simulink model "MdXX_RspChk"  (R2018b)
settings: Solver=FixedStepDiscrete  StartTime=0.0  StopTime=10.0  FixedStep=0.01  RelTol=1e-3
libraries: OutRspChkLib x20
(part 1 of 2)
settings Model: Creator=sn2xws  LastModifiedBy=sn2xws
settings DataIOCC: SaveFormat=StructureWithTime
settings OptimizationCC: DefaultParameterBehavior=Inlined  EnhancedBackFolding=on  PassReuseOutputArgsAs=Individual arguments  ZeroExternalMemoryAtStartup=off  ZeroInternalMemoryAtStartup=off  OptimizeBlockOrder=speed  DifferentSizesBufferReuse=on  OptimizationCustomize=off
settings DebuggingCC: ParameterTunabilityLossMsg=error
settings ModelReferenceCC: ModelReferenceNumInstancesAllowed=Single
settings SFSimCC: MATLABDynamicMemAlloc=off
settings RTWCC: SystemTargetFile=autosar.tlc  GenCodeOnly=on  TemplateMakefile=ert_default_tmf  Description=AUTOSAR  GenerateReport=on  IncludeHyperlinkInReport=on  LaunchReport=on  GenerateTraceInfo=on  GenerateTraceReport=on  GenerateTraceReportSl=on  GenerateTraceReportSf=on  GenerateTraceReportEml=on
settings CodeAppCC: ForceParamTrailComments=on  IgnoreCustomStorageClasses=off  OperatorAnnotations=on  SimulinkDataObjDesc=on  SFDataObjDesc=on  InsertBlockDesc=on
settings STFCustomTargetCC: TargetLangStandard=C99 (ISO)  MultiwordLength=256  ParMdlRefBuildCompliant=on  CompOptLevelCompliant=on  IncludeMdlTerminateFcn=off  CombineOutputUpdateFcns=on  SuppressErrorStatus=on  ERTCustomFileBanners=on  SupportNonFinite=off  SupportComplex=off  SupportContinuousTime=off  SupportNonInlinedSFcns=off  RemoveResetFunc=on  MATLABClassNameForMDSCustomization=Simulink.SoftwareTarget.ERTCustomization  AutosarCompliant=on  UseToolchainInfoCompliant=on  LookupTableObjectStructAxisOrder=2,1,3,4,...  LUTObjectStructOrderEvenSpacing=Size,Table,Breakpoints  SystemTargetFile=autosar.tlc
settings ERTTargetCC: TargetLangStandard=C99 (ISO)  ConcurrentExecutionCompliant=off  IncludeMdlTerminateFcn=off  SuppressErrorStatus=on  SupportNonFinite=off  SupportComplex=off  ModelStepFunctionPrototypeControlCompliant=off  CPPClassGenCompliant=off  AutosarCompliant=on  LookupTableObjectStructAxisOrder=2,1,3,4,...  LUTObjectStructOrderEvenSpacing=Size,Table,Breakpoints  InlinedParameterPlacement=NonHierarchical  ERTCustomFileTemplate=example_file_process.tlc

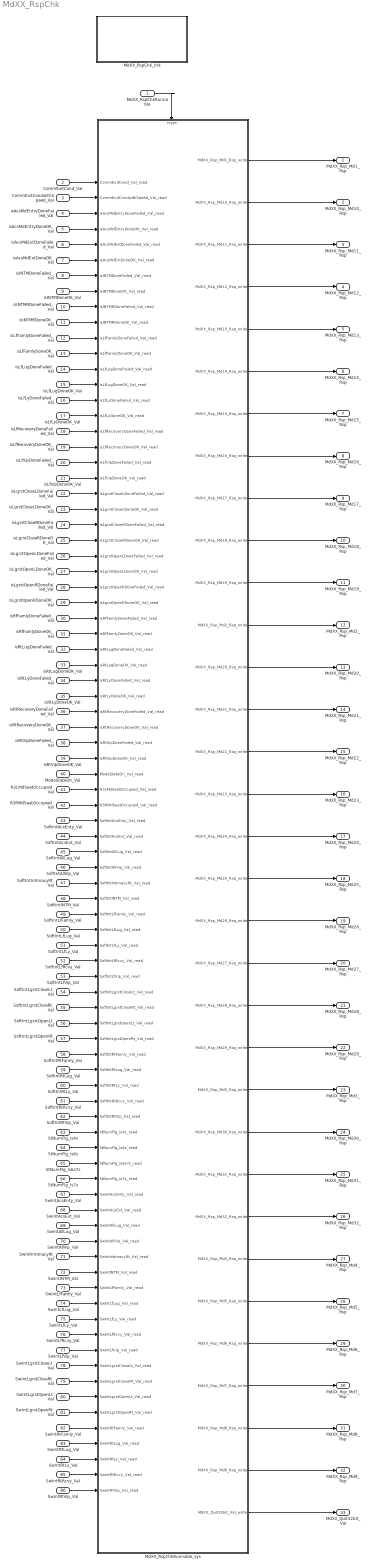
== system MdXX_RspChk ==
  MdXX_RspChkRunnable : Inport  SampleTime=0.01  OutputFunctionCall=on
  CommExitCond_Val : Inport  Port=2  OutDataTypeStr=boolean  PortDimensions=1
  CommExitCondwithSpeed_Val : Inport  Port=3  OutDataTypeStr=boolean  PortDimensions=1
  isAcsMdEntryDoneFailed_Val : Inport  Port=4  OutDataTypeStr=boolean  PortDimensions=1
  isAcsMdEntryDoneOK_Val : Inport  Port=5  OutDataTypeStr=boolean  PortDimensions=1
  isAcsMdExtDoneFailed_Val : Inport  Port=6  OutDataTypeStr=boolean  PortDimensions=1
  isAcsMdExtDoneOK_Val : Inport  Port=7  OutDataTypeStr=boolean  PortDimensions=1
  isINTMDoneFailed_Val : Inport  Port=8  OutDataTypeStr=boolean  PortDimensions=1
  isINTMDoneOK_Val : Inport  Port=9  OutDataTypeStr=boolean  PortDimensions=1
  isINTMRDoneFailed_Val : Inport  Port=10  OutDataTypeStr=boolean  PortDimensions=1
  isINTMRDoneOK_Val : Inport  Port=11  OutDataTypeStr=boolean  PortDimensions=1
  isLfFamlyDoneFailed_Val : Inport  Port=12  OutDataTypeStr=boolean  PortDimensions=1
  isLfFamlyDoneOK_Val : Inport  Port=13  OutDataTypeStr=boolean  PortDimensions=1
  isLfLugDoneFailed_Val : Inport  Port=14  OutDataTypeStr=boolean  PortDimensions=1
  isLfLugDoneOK_Val : Inport  Port=15  OutDataTypeStr=boolean  PortDimensions=1
  isLfLyDoneFailed_Val : Inport  Port=16  OutDataTypeStr=boolean  PortDimensions=1
  isLfLyDoneOK_Val : Inport  Port=17  OutDataTypeStr=boolean  PortDimensions=1
  isLfRecoveryDoneFailed_Val : Inport  Port=18  OutDataTypeStr=boolean  PortDimensions=1
  isLfRecoveryDoneOK_Val : Inport  Port=19  OutDataTypeStr=boolean  PortDimensions=1
  isLfVipDoneFailed_Val : Inport  Port=20  OutDataTypeStr=boolean  PortDimensions=1
  isLfVipDoneOK_Val : Inport  Port=21  OutDataTypeStr=boolean  PortDimensions=1
  isLgrstCloseLDoneFailed_Val : Inport  Port=22  OutDataTypeStr=boolean  PortDimensions=1
  isLgrstCloseLDoneOK_Val : Inport  Port=23  OutDataTypeStr=boolean  PortDimensions=1
  isLgrstCloseRDoneFailed_Val : Inport  Port=24  OutDataTypeStr=boolean  PortDimensions=1
  isLgrstCloseRDoneOK_Val : Inport  Port=25  OutDataTypeStr=boolean  PortDimensions=1
  isLgrstOpenLDoneFailed_Val : Inport  Port=26  OutDataTypeStr=boolean  PortDimensions=1
  isLgrstOpenLDoneOK_Val : Inport  Port=27  OutDataTypeStr=boolean  PortDimensions=1
  isLgrstOpenRDoneFailed_Val : Inport  Port=28  OutDataTypeStr=boolean  PortDimensions=1
  isLgrstOpenRDoneOK_Val : Inport  Port=29  OutDataTypeStr=boolean  PortDimensions=1
  isRfFamlyDoneFailed_Val : Inport  Port=30  OutDataTypeStr=boolean  PortDimensions=1
  isRfFamlyDoneOK_Val : Inport  Port=31  OutDataTypeStr=boolean  PortDimensions=1
  isRtLugDoneFailed_Val : Inport  Port=32  OutDataTypeStr=boolean  PortDimensions=1
  isRtLugDoneOK_Val : Inport  Port=33  OutDataTypeStr=boolean  PortDimensions=1
  isRtLyDoneFailed_Val : Inport  Port=34  OutDataTypeStr=boolean  PortDimensions=1
  isRtLyDoneOK_Val : Inport  Port=35  OutDataTypeStr=boolean  PortDimensions=1
  isRtRecoveryDoneFailed_Val : Inport  Port=36  OutDataTypeStr=boolean  PortDimensions=1
  isRtRecoveryDoneOK_Val : Inport  Port=37  OutDataTypeStr=boolean  PortDimensions=1
  isRtVipDoneFailed_Val : Inport  Port=38  OutDataTypeStr=boolean  PortDimensions=1
  isRtVipDoneOK_Val : Inport  Port=39  OutDataTypeStr=boolean  PortDimensions=1
  ModeStateOn_Val : Inport  Port=40  OutDataTypeStr=boolean  PortDimensions=1
  R3LMdSeatOccupied_Val : Inport  Port=41  OutDataTypeStr=boolean  PortDimensions=1
  R3RMdSeatOccupied_Val : Inport  Port=42  OutDataTypeStr=boolean  PortDimensions=1
  SoftIntAcsEnty_Val : Inport  Port=43  OutDataTypeStr=IntEnable  PortDimensions=1
  SoftIntAcsExt_Val : Inport  Port=44  OutDataTypeStr=IntEnable  PortDimensions=1
  SoftIntAllLug_Val : Inport  Port=45  OutDataTypeStr=IntEnable  PortDimensions=1
  SoftIntAllVip_Val : Inport  Port=46  OutDataTypeStr=IntEnable  PortDimensions=1
  SoftIntIntimacyRt_Val : Inport  Port=47  OutDataTypeStr=IntEnable  PortDimensions=1
  SoftIntINTM_Val : Inport  Port=48  OutDataTypeStr=IntEnable  PortDimensions=1
  SoftIntLfFamly_Val : Inport  Port=49  OutDataTypeStr=IntEnable  PortDimensions=1
  SoftIntLfLug_Val : Inport  Port=50  OutDataTypeStr=IntEnable  PortDimensions=1
  SoftIntLfLy_Val : Inport  Port=51  OutDataTypeStr=IntEnable  PortDimensions=1
  SoftIntLfRcvy_Val : Inport  Port=52  OutDataTypeStr=IntEnable  PortDimensions=1
  SoftIntLfVip_Val : Inport  Port=53  OutDataTypeStr=IntEnable  PortDimensions=1
  SoftIntLgrstCloseLt_Val : Inport  Port=54  OutDataTypeStr=IntEnable  PortDimensions=1
  SoftIntLgrstCloseRt_Val : Inport  Port=55  OutDataTypeStr=IntEnable  PortDimensions=1
  SoftIntLgrstOpenLt_Val : Inport  Port=56  OutDataTypeStr=IntEnable  PortDimensions=1
  SoftIntLgrstOpenRt_Val : Inport  Port=57  OutDataTypeStr=IntEnable  PortDimensions=1
  SoftIntRtFamly_Val : Inport  Port=58  OutDataTypeStr=IntEnable  PortDimensions=1
  SoftIntRtLug_Val : Inport  Port=59  OutDataTypeStr=IntEnable  PortDimensions=1
  SoftIntRtLy_Val : Inport  Port=60  OutDataTypeStr=IntEnable  PortDimensions=1
  SoftIntRtRcvy_Val : Inport  Port=61  OutDataTypeStr=IntEnable  PortDimensions=1
  SoftIntRtVip_Val : Inport  Port=62  OutDataTypeStr=IntEnable  PortDimensions=1
  StNumFlg_Is4s : Inport  Port=63  OutDataTypeStr=boolean  PortDimensions=1
  StNumFlg_Is6s : Inport  Port=64  OutDataTypeStr=boolean  PortDimensions=1
  StNumFlg_Is6s7s : Inport  Port=65  OutDataTypeStr=boolean  PortDimensions=1
  StNumFlg_Is7s : Inport  Port=66  OutDataTypeStr=boolean  PortDimensions=1
  SwIntAcsEnty_Val : Inport  Port=67  OutDataTypeStr=IntEnable  PortDimensions=1
  SwIntAcsExt_Val : Inport  Port=68  OutDataTypeStr=IntEnable  PortDimensions=1
  SwIntAllLug_Val : Inport  Port=69  OutDataTypeStr=IntEnable  PortDimensions=1
  SwIntAllVip_Val : Inport  Port=70  OutDataTypeStr=IntEnable  PortDimensions=1
  SwIntIntimacyRt_Val : Inport  Port=71  OutDataTypeStr=IntEnable  PortDimensions=1
  SwIntINTM_Val : Inport  Port=72  OutDataTypeStr=IntEnable  PortDimensions=1
  SwIntLfFamly_Val : Inport  Port=73  OutDataTypeStr=IntEnable  PortDimensions=1
  SwIntLfLug_Val : Inport  Port=74  OutDataTypeStr=IntEnable  PortDimensions=1
  SwIntLfLy_Val : Inport  Port=75  OutDataTypeStr=IntEnable  PortDimensions=1
  SwIntLfRcvy_Val : Inport  Port=76  OutDataTypeStr=IntEnable  PortDimensions=1
  SwIntLfVip_Val : Inport  Port=77  OutDataTypeStr=IntEnable  PortDimensions=1
  SwIntLgrstCloseLt_Val : Inport  Port=78  OutDataTypeStr=IntEnable  PortDimensions=1
  SwIntLgrstCloseRt_Val : Inport  Port=79  OutDataTypeStr=IntEnable  PortDimensions=1
  SwIntLgrstOpenLt_Val : Inport  Port=80  OutDataTypeStr=IntEnable  PortDimensions=1
  SwIntLgrstOpenRt_Val : Inport  Port=81  OutDataTypeStr=IntEnable  PortDimensions=1
  SwIntRtFamly_Val : Inport  Port=82  OutDataTypeStr=IntEnable  PortDimensions=1
  SwIntRtLug_Val : Inport  Port=83  OutDataTypeStr=IntEnable  PortDimensions=1
  SwIntRtLy_Val : Inport  Port=84  OutDataTypeStr=IntEnable  PortDimensions=1
  SwIntRtRcvy_Val : Inport  Port=85  OutDataTypeStr=IntEnable  PortDimensions=1
  SwIntRtVip_Val : Inport  Port=86  OutDataTypeStr=IntEnable  PortDimensions=1
  MdXX_RspChkRunnable_sys : Subsystem
  MdXX_RspChk_Init : Subsystem
  MdXX_Rsp_Md1_Rsp : Outport  OutDataTypeStr=Enum: MdRspLocal2  PortDimensions=1
  MdXX_Rsp_Md10_Rsp : Outport  Port=2  OutDataTypeStr=Enum: MdRspLocal2  PortDimensions=1
  MdXX_Rsp_Md11_Rsp : Outport  Port=3  OutDataTypeStr=Enum: MdRspLocal2  PortDimensions=1
  MdXX_Rsp_Md12_Rsp : Outport  Port=4  OutDataTypeStr=Enum: MdRspLocal2  PortDimensions=1
  MdXX_Rsp_Md13_Rsp : Outport  Port=5  OutDataTypeStr=Enum: MdRspLocal2  PortDimensions=1
  MdXX_Rsp_Md14_Rsp : Outport  Port=6  OutDataTypeStr=Enum: MdRspLocal2  PortDimensions=1
  MdXX_Rsp_Md15_Rsp : Outport  Port=7  OutDataTypeStr=Enum: MdRspLocal2  PortDimensions=1
  MdXX_Rsp_Md16_Rsp : Outport  Port=8  OutDataTypeStr=Enum: MdRspLocal2  PortDimensions=1
  MdXX_Rsp_Md17_Rsp : Outport  Port=9  OutDataTypeStr=Enum: MdRspLocal2  PortDimensions=1
  MdXX_Rsp_Md18_Rsp : Outport  Port=10  OutDataTypeStr=Enum: MdRspLocal2  PortDimensions=1
  MdXX_Rsp_Md19_Rsp : Outport  Port=11  OutDataTypeStr=Enum: MdRspLocal2  PortDimensions=1
  MdXX_Rsp_Md2_Rsp : Outport  Port=12  OutDataTypeStr=Enum: MdRspLocal2  PortDimensions=1
  MdXX_Rsp_Md20_Rsp : Outport  Port=13  OutDataTypeStr=Enum: MdRspLocal2  PortDimensions=1
  MdXX_Rsp_Md21_Rsp : Outport  Port=14  OutDataTypeStr=Enum: MdRspLocal2  PortDimensions=1
  MdXX_Rsp_Md22_Rsp : Outport  Port=15  OutDataTypeStr=Enum: MdRspLocal2  PortDimensions=1
  MdXX_Rsp_Md23_Rsp : Outport  Port=16  OutDataTypeStr=Enum: MdRspLocal2  PortDimensions=1
  MdXX_Rsp_Md24_Rsp : Outport  Port=17  OutDataTypeStr=Enum: MdRspLocal2  PortDimensions=1
  MdXX_Rsp_Md25_Rsp : Outport  Port=18  OutDataTypeStr=Enum: MdRspLocal2  PortDimensions=1
  MdXX_Rsp_Md26_Rsp : Outport  Port=19  OutDataTypeStr=Enum: MdRspLocal2  PortDimensions=1
  MdXX_Rsp_Md27_Rsp : Outport  Port=20  OutDataTypeStr=Enum: MdRspLocal2  PortDimensions=1
  MdXX_Rsp_Md28_Rsp : Outport  Port=21  OutDataTypeStr=Enum: MdRspLocal2  PortDimensions=1
  MdXX_Rsp_Md29_Rsp : Outport  Port=22  OutDataTypeStr=Enum: MdRspLocal2  PortDimensions=1
  MdXX_Rsp_Md3_Rsp : Outport  Port=23  OutDataTypeStr=Enum: MdRspLocal2  PortDimensions=1
  MdXX_Rsp_Md30_Rsp : Outport  Port=24  OutDataTypeStr=Enum: MdRspLocal2  PortDimensions=1
  MdXX_Rsp_Md31_Rsp : Outport  Port=25  OutDataTypeStr=Enum: MdRspLocal2  PortDimensions=1
  MdXX_Rsp_Md32_Rsp : Outport  Port=26  OutDataTypeStr=Enum: MdRspLocal2  PortDimensions=1
  MdXX_Rsp_Md4_Rsp : Outport  Port=27  OutDataTypeStr=Enum: MdRspLocal2  PortDimensions=1
  MdXX_Rsp_Md5_Rsp : Outport  Port=28  OutDataTypeStr=Enum: MdRspLocal2  PortDimensions=1
  MdXX_Rsp_Md6_Rsp : Outport  Port=29  OutDataTypeStr=Enum: MdRspLocal2  PortDimensions=1
  MdXX_Rsp_Md7_Rsp : Outport  Port=30  OutDataTypeStr=Enum: MdRspLocal2  PortDimensions=1
  MdXX_Rsp_Md8_Rsp : Outport  Port=31  OutDataTypeStr=Enum: MdRspLocal2  PortDimensions=1
  MdXX_Rsp_Md9_Rsp : Outport  Port=32  OutDataTypeStr=Enum: MdRspLocal2  PortDimensions=1
  MdXX_Quit32bit_Val : Outport  Port=33  OutDataTypeStr=uint32  PortDimensions=1
  wires:
  CommExitCond_Val/1 -> MdXX_RspChkRunnable_sys/1(CommExitCond_Val_read)
  CommExitCondwithSpeed_Val/1 -> MdXX_RspChkRunnable_sys/2(CommExitCondwithSpeed_Val_read)
  isAcsMdEntryDoneFailed_Val/1 -> MdXX_RspChkRunnable_sys/3(isAcsMdEntryDoneFailed_Val_read)
  isAcsMdEntryDoneOK_Val/1 -> MdXX_RspChkRunnable_sys/4(isAcsMdEntryDoneOK_Val_read)
  isAcsMdExtDoneFailed_Val/1 -> MdXX_RspChkRunnable_sys/5(isAcsMdExtDoneFailed_Val_read)
  isAcsMdExtDoneOK_Val/1 -> MdXX_RspChkRunnable_sys/6(isAcsMdExtDoneOK_Val_read)
  isINTMDoneFailed_Val/1 -> MdXX_RspChkRunnable_sys/7(isINTMDoneFailed_Val_read)
  isINTMDoneOK_Val/1 -> MdXX_RspChkRunnable_sys/8(isINTMDoneOK_Val_read)
  isINTMRDoneFailed_Val/1 -> MdXX_RspChkRunnable_sys/9(isINTMRDoneFailed_Val_read)
  isINTMRDoneOK_Val/1 -> MdXX_RspChkRunnable_sys/10(isINTMRDoneOK_Val_read)
  isLfFamlyDoneFailed_Val/1 -> MdXX_RspChkRunnable_sys/11(isLfFamlyDoneFailed_Val_read)
  isLfFamlyDoneOK_Val/1 -> MdXX_RspChkRunnable_sys/12(isLfFamlyDoneOK_Val_read)
  isLfLugDoneFailed_Val/1 -> MdXX_RspChkRunnable_sys/13(isLfLugDoneFailed_Val_read)
  isLfLugDoneOK_Val/1 -> MdXX_RspChkRunnable_sys/14(isLfLugDoneOK_Val_read)
  isLfLyDoneFailed_Val/1 -> MdXX_RspChkRunnable_sys/15(isLfLyDoneFailed_Val_read)
  isLfLyDoneOK_Val/1 -> MdXX_RspChkRunnable_sys/16(isLfLyDoneOK_Val_read)
  isLfRecoveryDoneFailed_Val/1 -> MdXX_RspChkRunnable_sys/17(isLfRecoveryDoneFailed_Val_read)
  isLfRecoveryDoneOK_Val/1 -> MdXX_RspChkRunnable_sys/18(isLfRecoveryDoneOK_Val_read)
  isLfVipDoneFailed_Val/1 -> MdXX_RspChkRunnable_sys/19(isLfVipDoneFailed_Val_read)
  isLfVipDoneOK_Val/1 -> MdXX_RspChkRunnable_sys/20(isLfVipDoneOK_Val_read)
  isLgrstCloseLDoneFailed_Val/1 -> MdXX_RspChkRunnable_sys/21(isLgrstCloseLDoneFailed_Val_read)
  isLgrstCloseLDoneOK_Val/1 -> MdXX_RspChkRunnable_sys/22(isLgrstCloseLDoneOK_Val_read)
  isLgrstCloseRDoneFailed_Val/1 -> MdXX_RspChkRunnable_sys/23(isLgrstCloseRDoneFailed_Val_read)
  isLgrstCloseRDoneOK_Val/1 -> MdXX_RspChkRunnable_sys/24(isLgrstCloseRDoneOK_Val_read)
  isLgrstOpenLDoneFailed_Val/1 -> MdXX_RspChkRunnable_sys/25(isLgrstOpenLDoneFailed_Val_read)
  isLgrstOpenLDoneOK_Val/1 -> MdXX_RspChkRunnable_sys/26(isLgrstOpenLDoneOK_Val_read)
  isLgrstOpenRDoneFailed_Val/1 -> MdXX_RspChkRunnable_sys/27(isLgrstOpenRDoneFailed_Val_read)
  isLgrstOpenRDoneOK_Val/1 -> MdXX_RspChkRunnable_sys/28(isLgrstOpenRDoneOK_Val_read)
  isRfFamlyDoneFailed_Val/1 -> MdXX_RspChkRunnable_sys/29(isRfFamlyDoneFailed_Val_read)
  isRfFamlyDoneOK_Val/1 -> MdXX_RspChkRunnable_sys/30(isRfFamlyDoneOK_Val_read)
  isRtLugDoneFailed_Val/1 -> MdXX_RspChkRunnable_sys/31(isRtLugDoneFailed_Val_read)
  isRtLugDoneOK_Val/1 -> MdXX_RspChkRunnable_sys/32(isRtLugDoneOK_Val_read)
  isRtLyDoneFailed_Val/1 -> MdXX_RspChkRunnable_sys/33(isRtLyDoneFailed_Val_read)
  isRtLyDoneOK_Val/1 -> MdXX_RspChkRunnable_sys/34(isRtLyDoneOK_Val_read)
  isRtRecoveryDoneFailed_Val/1 -> MdXX_RspChkRunnable_sys/35(isRtRecoveryDoneFailed_Val_read)
  isRtRecoveryDoneOK_Val/1 -> MdXX_RspChkRunnable_sys/36(isRtRecoveryDoneOK_Val_read)
  isRtVipDoneFailed_Val/1 -> MdXX_RspChkRunnable_sys/37(isRtVipDoneFailed_Val_read)
  isRtVipDoneOK_Val/1 -> MdXX_RspChkRunnable_sys/38(isRtVipDoneOK_Val_read)
  ModeStateOn_Val/1 -> MdXX_RspChkRunnable_sys/39(ModeStateOn_Val_read)
  R3LMdSeatOccupied_Val/1 -> MdXX_RspChkRunnable_sys/40(R3LMdSeatOccupied_Val_read)
  R3RMdSeatOccupied_Val/1 -> MdXX_RspChkRunnable_sys/41(R3RMdSeatOccupied_Val_read)
  SoftIntAcsEnty_Val/1 -> MdXX_RspChkRunnable_sys/42(SoftIntAcsEnty_Val_read)
  SoftIntAcsExt_Val/1 -> MdXX_RspChkRunnable_sys/43(SoftIntAcsExt_Val_read)
  SoftIntAllLug_Val/1 -> MdXX_RspChkRunnable_sys/44(SoftIntAllLug_Val_read)
  SoftIntAllVip_Val/1 -> MdXX_RspChkRunnable_sys/45(SoftIntAllVip_Val_read)
  SoftIntIntimacyRt_Val/1 -> MdXX_RspChkRunnable_sys/46(SoftIntIntimacyRt_Val_read)
  SoftIntINTM_Val/1 -> MdXX_RspChkRunnable_sys/47(SoftIntINTM_Val_read)
  SoftIntLfFamly_Val/1 -> MdXX_RspChkRunnable_sys/48(SoftIntLfFamly_Val_read)
  SoftIntLfLug_Val/1 -> MdXX_RspChkRunnable_sys/49(SoftIntLfLug_Val_read)
  SoftIntLfLy_Val/1 -> MdXX_RspChkRunnable_sys/50(SoftIntLfLy_Val_read)
  SoftIntLfRcvy_Val/1 -> MdXX_RspChkRunnable_sys/51(SoftIntLfRcvy_Val_read)
  SoftIntLfVip_Val/1 -> MdXX_RspChkRunnable_sys/52(SoftIntLfVip_Val_read)
  SoftIntLgrstCloseLt_Val/1 -> MdXX_RspChkRunnable_sys/53(SoftIntLgrstCloseLt_Val_read)
  SoftIntLgrstCloseRt_Val/1 -> MdXX_RspChkRunnable_sys/54(SoftIntLgrstCloseRt_Val_read)
  SoftIntLgrstOpenLt_Val/1 -> MdXX_RspChkRunnable_sys/55(SoftIntLgrstOpenLt_Val_read)
  SoftIntLgrstOpenRt_Val/1 -> MdXX_RspChkRunnable_sys/56(SoftIntLgrstOpenRt_Val_read)
  SoftIntRtFamly_Val/1 -> MdXX_RspChkRunnable_sys/57(SoftIntRtFamly_Val_read)
  SoftIntRtLug_Val/1 -> MdXX_RspChkRunnable_sys/58(SoftIntRtLug_Val_read)
  SoftIntRtLy_Val/1 -> MdXX_RspChkRunnable_sys/59(SoftIntRtLy_Val_read)
  SoftIntRtRcvy_Val/1 -> MdXX_RspChkRunnable_sys/60(SoftIntRtRcvy_Val_read)
  SoftIntRtVip_Val/1 -> MdXX_RspChkRunnable_sys/61(SoftIntRtVip_Val_read)
  StNumFlg_Is4s/1 -> MdXX_RspChkRunnable_sys/62(StNumFlg_Is4s_read)
  StNumFlg_Is6s/1 -> MdXX_RspChkRunnable_sys/63(StNumFlg_Is6s_read)
  StNumFlg_Is6s7s/1 -> MdXX_RspChkRunnable_sys/64(StNumFlg_Is6s7s_read)
  StNumFlg_Is7s/1 -> MdXX_RspChkRunnable_sys/65(StNumFlg_Is7s_read)
  SwIntAcsEnty_Val/1 -> MdXX_RspChkRunnable_sys/66(SwIntAcsEnty_Val_read)
  SwIntAcsExt_Val/1 -> MdXX_RspChkRunnable_sys/67(SwIntAcsExt_Val_read)
  SwIntAllLug_Val/1 -> MdXX_RspChkRunnable_sys/68(SwIntAllLug_Val_read)
  SwIntAllVip_Val/1 -> MdXX_RspChkRunnable_sys/69(SwIntAllVip_Val_read)
  SwIntIntimacyRt_Val/1 -> MdXX_RspChkRunnable_sys/70(SwIntIntimacyRt_Val_read)
  SwIntINTM_Val/1 -> MdXX_RspChkRunnable_sys/71(SwIntINTM_Val_read)
  SwIntLfFamly_Val/1 -> MdXX_RspChkRunnable_sys/72(SwIntLfFamly_Val_read)
  SwIntLfLug_Val/1 -> MdXX_RspChkRunnable_sys/73(SwIntLfLug_Val_read)
  SwIntLfLy_Val/1 -> MdXX_RspChkRunnable_sys/74(SwIntLfLy_Val_read)
  SwIntLfRcvy_Val/1 -> MdXX_RspChkRunnable_sys/75(SwIntLfRcvy_Val_read)
  SwIntLfVip_Val/1 -> MdXX_RspChkRunnable_sys/76(SwIntLfVip_Val_read)
  SwIntLgrstCloseLt_Val/1 -> MdXX_RspChkRunnable_sys/77(SwIntLgrstCloseLt_Val_read)
  SwIntLgrstCloseRt_Val/1 -> MdXX_RspChkRunnable_sys/78(SwIntLgrstCloseRt_Val_read)
  SwIntLgrstOpenLt_Val/1 -> MdXX_RspChkRunnable_sys/79(SwIntLgrstOpenLt_Val_read)
  SwIntLgrstOpenRt_Val/1 -> MdXX_RspChkRunnable_sys/80(SwIntLgrstOpenRt_Val_read)
  SwIntRtFamly_Val/1 -> MdXX_RspChkRunnable_sys/81(SwIntRtFamly_Val_read)
  SwIntRtLug_Val/1 -> MdXX_RspChkRunnable_sys/82(SwIntRtLug_Val_read)
  SwIntRtLy_Val/1 -> MdXX_RspChkRunnable_sys/83(SwIntRtLy_Val_read)
  SwIntRtRcvy_Val/1 -> MdXX_RspChkRunnable_sys/84(SwIntRtRcvy_Val_read)
  SwIntRtVip_Val/1 -> MdXX_RspChkRunnable_sys/85(SwIntRtVip_Val_read)
  MdXX_RspChkRunnable_sys/1(MdXX_Rsp_Md1_Rsp_write) -> MdXX_Rsp_Md1_Rsp/1
  MdXX_RspChkRunnable_sys/2(MdXX_Rsp_Md10_Rsp_write) -> MdXX_Rsp_Md10_Rsp/1
  MdXX_RspChkRunnable_sys/3(MdXX_Rsp_Md11_Rsp_write) -> MdXX_Rsp_Md11_Rsp/1
  MdXX_RspChkRunnable_sys/4(MdXX_Rsp_Md12_Rsp_write) -> MdXX_Rsp_Md12_Rsp/1
  MdXX_RspChkRunnable_sys/5(MdXX_Rsp_Md13_Rsp_write) -> MdXX_Rsp_Md13_Rsp/1
  MdXX_RspChkRunnable_sys/6(MdXX_Rsp_Md14_Rsp_write) -> MdXX_Rsp_Md14_Rsp/1
  MdXX_RspChkRunnable_sys/7(MdXX_Rsp_Md15_Rsp_write) -> MdXX_Rsp_Md15_Rsp/1
  MdXX_RspChkRunnable_sys/8(MdXX_Rsp_Md16_Rsp_write) -> MdXX_Rsp_Md16_Rsp/1
  MdXX_RspChkRunnable_sys/9(MdXX_Rsp_Md17_Rsp_write) -> MdXX_Rsp_Md17_Rsp/1
  MdXX_RspChkRunnable_sys/10(MdXX_Rsp_Md18_Rsp_write) -> MdXX_Rsp_Md18_Rsp/1
  MdXX_RspChkRunnable_sys/11(MdXX_Rsp_Md19_Rsp_write) -> MdXX_Rsp_Md19_Rsp/1
  MdXX_RspChkRunnable_sys/12(MdXX_Rsp_Md2_Rsp_write) -> MdXX_Rsp_Md2_Rsp/1
  MdXX_RspChkRunnable_sys/13(MdXX_Rsp_Md20_Rsp_write) -> MdXX_Rsp_Md20_Rsp/1
  MdXX_RspChkRunnable_sys/14(MdXX_Rsp_Md21_Rsp_write) -> MdXX_Rsp_Md21_Rsp/1
  MdXX_RspChkRunnable_sys/15(MdXX_Rsp_Md22_Rsp_write) -> MdXX_Rsp_Md22_Rsp/1
  MdXX_RspChkRunnable_sys/16(MdXX_Rsp_Md23_Rsp_write) -> MdXX_Rsp_Md23_Rsp/1
  MdXX_RspChkRunnable_sys/17(MdXX_Rsp_Md24_Rsp_write) -> MdXX_Rsp_Md24_Rsp/1
  MdXX_RspChkRunnable_sys/18(MdXX_Rsp_Md25_Rsp_write) -> MdXX_Rsp_Md25_Rsp/1
  MdXX_RspChkRunnable_sys/19(MdXX_Rsp_Md26_Rsp_write) -> MdXX_Rsp_Md26_Rsp/1
  MdXX_RspChkRunnable_sys/20(MdXX_Rsp_Md27_Rsp_write) -> MdXX_Rsp_Md27_Rsp/1
  MdXX_RspChkRunnable_sys/21(MdXX_Rsp_Md28_Rsp_write) -> MdXX_Rsp_Md28_Rsp/1
  MdXX_RspChkRunnable_sys/22(MdXX_Rsp_Md29_Rsp_write) -> MdXX_Rsp_Md29_Rsp/1
  MdXX_RspChkRunnable_sys/23(MdXX_Rsp_Md3_Rsp_write) -> MdXX_Rsp_Md3_Rsp/1
  MdXX_RspChkRunnable_sys/24(MdXX_Rsp_Md30_Rsp_write) -> MdXX_Rsp_Md30_Rsp/1
  MdXX_RspChkRunnable_sys/25(MdXX_Rsp_Md31_Rsp_write) -> MdXX_Rsp_Md31_Rsp/1
  MdXX_RspChkRunnable_sys/26(MdXX_Rsp_Md32_Rsp_write) -> MdXX_Rsp_Md32_Rsp/1
  MdXX_RspChkRunnable_sys/27(MdXX_Rsp_Md4_Rsp_write) -> MdXX_Rsp_Md4_Rsp/1
  MdXX_RspChkRunnable_sys/28(MdXX_Rsp_Md5_Rsp_write) -> MdXX_Rsp_Md5_Rsp/1
  MdXX_RspChkRunnable_sys/29(MdXX_Rsp_Md6_Rsp_write) -> MdXX_Rsp_Md6_Rsp/1
  MdXX_RspChkRunnable_sys/30(MdXX_Rsp_Md7_Rsp_write) -> MdXX_Rsp_Md7_Rsp/1
  MdXX_RspChkRunnable_sys/31(MdXX_Rsp_Md8_Rsp_write) -> MdXX_Rsp_Md8_Rsp/1
  MdXX_RspChkRunnable_sys/32(MdXX_Rsp_Md9_Rsp_write) -> MdXX_Rsp_Md9_Rsp/1
  MdXX_RspChkRunnable_sys/33(MdXX_Quit32bit_Val_write) -> MdXX_Quit32bit_Val/1
  MdXX_RspChkRunnable/1 -> MdXX_RspChkRunnable_sys/Trigger

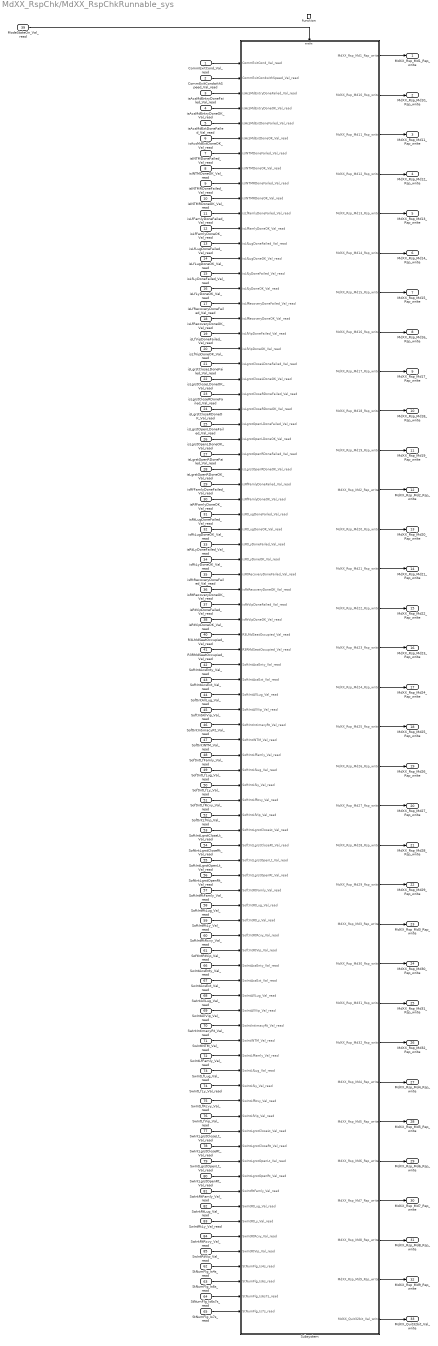
== system MdXX_RspChk/MdXX_RspChkRunnable_sys ==
  CommExitCond_Val_read : Inport
  CommExitCondwithSpeed_Val_read : Inport  Port=2
  isAcsMdEntryDoneFailed_Val_read : Inport  Port=3
  isAcsMdEntryDoneOK_Val_read : Inport  Port=4
  isAcsMdExtDoneFailed_Val_read : Inport  Port=5
  isAcsMdExtDoneOK_Val_read : Inport  Port=6
  isINTMDoneFailed_Val_read : Inport  Port=7
  isINTMDoneOK_Val_read : Inport  Port=8
  isINTMRDoneFailed_Val_read : Inport  Port=9
  isINTMRDoneOK_Val_read : Inport  Port=10
  isLfFamlyDoneFailed_Val_read : Inport  Port=11
  isLfFamlyDoneOK_Val_read : Inport  Port=12
  isLfLugDoneFailed_Val_read : Inport  Port=13
  isLfLugDoneOK_Val_read : Inport  Port=14
  isLfLyDoneFailed_Val_read : Inport  Port=15
  isLfLyDoneOK_Val_read : Inport  Port=16
  isLfRecoveryDoneFailed_Val_read : Inport  Port=17
  isLfRecoveryDoneOK_Val_read : Inport  Port=18
  isLfVipDoneFailed_Val_read : Inport  Port=19
  isLfVipDoneOK_Val_read : Inport  Port=20
  isLgrstCloseLDoneFailed_Val_read : Inport  Port=21
  isLgrstCloseLDoneOK_Val_read : Inport  Port=22
  isLgrstCloseRDoneFailed_Val_read : Inport  Port=23
  isLgrstCloseRDoneOK_Val_read : Inport  Port=24
  isLgrstOpenLDoneFailed_Val_read : Inport  Port=25
  isLgrstOpenLDoneOK_Val_read : Inport  Port=26
  isLgrstOpenRDoneFailed_Val_read : Inport  Port=27
  isLgrstOpenRDoneOK_Val_read : Inport  Port=28
  isRfFamlyDoneFailed_Val_read : Inport  Port=29
  isRfFamlyDoneOK_Val_read : Inport  Port=30
  isRtLugDoneFailed_Val_read : Inport  Port=31
  isRtLugDoneOK_Val_read : Inport  Port=32
  isRtLyDoneFailed_Val_read : Inport  Port=33
  isRtLyDoneOK_Val_read : Inport  Port=34
  isRtRecoveryDoneFailed_Val_read : Inport  Port=35
  isRtRecoveryDoneOK_Val_read : Inport  Port=36
  isRtVipDoneFailed_Val_read : Inport  Port=37
  isRtVipDoneOK_Val_read : Inport  Port=38
  ModeStateOn_Val_read : Inport  Port=39
  R3LMdSeatOccupied_Val_read : Inport  Port=40
  R3RMdSeatOccupied_Val_read : Inport  Port=41
  SoftIntAcsEnty_Val_read : Inport  Port=42
  SoftIntAcsExt_Val_read : Inport  Port=43
  SoftIntAllLug_Val_read : Inport  Port=44
  SoftIntAllVip_Val_read : Inport  Port=45
  SoftIntIntimacyRt_Val_read : Inport  Port=46
  SoftIntINTM_Val_read : Inport  Port=47
  SoftIntLfFamly_Val_read : Inport  Port=48
  SoftIntLfLug_Val_read : Inport  Port=49
  SoftIntLfLy_Val_read : Inport  Port=50
  SoftIntLfRcvy_Val_read : Inport  Port=51
  SoftIntLfVip_Val_read : Inport  Port=52
  SoftIntLgrstCloseLt_Val_read : Inport  Port=53
  SoftIntLgrstCloseRt_Val_read : Inport  Port=54
  SoftIntLgrstOpenLt_Val_read : Inport  Port=55
  SoftIntLgrstOpenRt_Val_read : Inport  Port=56
  SoftIntRtFamly_Val_read : Inport  Port=57
  SoftIntRtLug_Val_read : Inport  Port=58
  SoftIntRtLy_Val_read : Inport  Port=59
  SoftIntRtRcvy_Val_read : Inport  Port=60
  SoftIntRtVip_Val_read : Inport  Port=61
  StNumFlg_Is4s_read : Inport  Port=62
  StNumFlg_Is6s_read : Inport  Port=63
  StNumFlg_Is6s7s_read : Inport  Port=64
  StNumFlg_Is7s_read : Inport  Port=65
  SwIntAcsEnty_Val_read : Inport  Port=66
  SwIntAcsExt_Val_read : Inport  Port=67
  SwIntAllLug_Val_read : Inport  Port=68
  SwIntAllVip_Val_read : Inport  Port=69
  SwIntIntimacyRt_Val_read : Inport  Port=70
  SwIntINTM_Val_read : Inport  Port=71
  SwIntLfFamly_Val_read : Inport  Port=72
  SwIntLfLug_Val_read : Inport  Port=73
  SwIntLfLy_Val_read : Inport  Port=74
  SwIntLfRcvy_Val_read : Inport  Port=75
  SwIntLfVip_Val_read : Inport  Port=76
  SwIntLgrstCloseLt_Val_read : Inport  Port=77
  SwIntLgrstCloseRt_Val_read : Inport  Port=78
  SwIntLgrstOpenLt_Val_read : Inport  Port=79
  SwIntLgrstOpenRt_Val_read : Inport  Port=80
  SwIntRtFamly_Val_read : Inport  Port=81
  SwIntRtLug_Val_read : Inport  Port=82
  SwIntRtLy_Val_read : Inport  Port=83
  SwIntRtRcvy_Val_read : Inport  Port=84
  SwIntRtVip_Val_read : Inport  Port=85
  function : TriggerPort  TriggerType=function-call  VariantControl=(inherit)  SampleTimeType=periodic  SampleTime=-1
  Subsystem : Subsystem
  MdXX_Rsp_Md1_Rsp_write : Outport
      settings: EnsureOutportIsVirtual=on
  MdXX_Rsp_Md10_Rsp_write : Outport  Port=2
      settings: EnsureOutportIsVirtual=on
  MdXX_Rsp_Md11_Rsp_write : Outport  Port=3
      settings: EnsureOutportIsVirtual=on
  MdXX_Rsp_Md12_Rsp_write : Outport  Port=4
      settings: EnsureOutportIsVirtual=on
  MdXX_Rsp_Md13_Rsp_write : Outport  Port=5
      settings: EnsureOutportIsVirtual=on
  MdXX_Rsp_Md14_Rsp_write : Outport  Port=6
      settings: EnsureOutportIsVirtual=on
  MdXX_Rsp_Md15_Rsp_write : Outport  Port=7
      settings: EnsureOutportIsVirtual=on
  MdXX_Rsp_Md16_Rsp_write : Outport  Port=8
      settings: EnsureOutportIsVirtual=on
  MdXX_Rsp_Md17_Rsp_write : Outport  Port=9
      settings: EnsureOutportIsVirtual=on
  MdXX_Rsp_Md18_Rsp_write : Outport  Port=10
      settings: EnsureOutportIsVirtual=on
  MdXX_Rsp_Md19_Rsp_write : Outport  Port=11
      settings: EnsureOutportIsVirtual=on
  MdXX_Rsp_Md2_Rsp_write : Outport  Port=12
      settings: EnsureOutportIsVirtual=on
  MdXX_Rsp_Md20_Rsp_write : Outport  Port=13
      settings: EnsureOutportIsVirtual=on
  MdXX_Rsp_Md21_Rsp_write : Outport  Port=14
      settings: EnsureOutportIsVirtual=on
  MdXX_Rsp_Md22_Rsp_write : Outport  Port=15
      settings: EnsureOutportIsVirtual=on
  MdXX_Rsp_Md23_Rsp_write : Outport  Port=16
      settings: EnsureOutportIsVirtual=on
  MdXX_Rsp_Md24_Rsp_write : Outport  Port=17
      settings: EnsureOutportIsVirtual=on
  MdXX_Rsp_Md25_Rsp_write : Outport  Port=18
      settings: EnsureOutportIsVirtual=on
  MdXX_Rsp_Md26_Rsp_write : Outport  Port=19
      settings: EnsureOutportIsVirtual=on
  MdXX_Rsp_Md27_Rsp_write : Outport  Port=20
      settings: EnsureOutportIsVirtual=on
  MdXX_Rsp_Md28_Rsp_write : Outport  Port=21
      settings: EnsureOutportIsVirtual=on
  MdXX_Rsp_Md29_Rsp_write : Outport  Port=22
      settings: EnsureOutportIsVirtual=on
  MdXX_Rsp_Md3_Rsp_write : Outport  Port=23
      settings: EnsureOutportIsVirtual=on
  MdXX_Rsp_Md30_Rsp_write : Outport  Port=24
      settings: EnsureOutportIsVirtual=on
  MdXX_Rsp_Md31_Rsp_write : Outport  Port=25
      settings: EnsureOutportIsVirtual=on
  MdXX_Rsp_Md32_Rsp_write : Outport  Port=26
      settings: EnsureOutportIsVirtual=on
  MdXX_Rsp_Md4_Rsp_write : Outport  Port=27
      settings: EnsureOutportIsVirtual=on
  MdXX_Rsp_Md5_Rsp_write : Outport  Port=28
      settings: EnsureOutportIsVirtual=on
  MdXX_Rsp_Md6_Rsp_write : Outport  Port=29
      settings: EnsureOutportIsVirtual=on
  MdXX_Rsp_Md7_Rsp_write : Outport  Port=30
      settings: EnsureOutportIsVirtual=on
  MdXX_Rsp_Md8_Rsp_write : Outport  Port=31
      settings: EnsureOutportIsVirtual=on
  MdXX_Rsp_Md9_Rsp_write : Outport  Port=32
      settings: EnsureOutportIsVirtual=on
  MdXX_Quit32bit_Val_write : Outport  Port=33
      settings: EnsureOutportIsVirtual=on
  wires:
  ModeStateOn_Val_read/1 -> Subsystem/Enable
  CommExitCond_Val_read/1 -> Subsystem/1(CommExitCond_Val_read)
  CommExitCondwithSpeed_Val_read/1 -> Subsystem/2(CommExitCondwithSpeed_Val_read)
  isAcsMdEntryDoneFailed_Val_read/1 -> Subsystem/3(isAcsMdEntryDoneFailed_Val_read)
  isAcsMdEntryDoneOK_Val_read/1 -> Subsystem/4(isAcsMdEntryDoneOK_Val_read)
  isAcsMdExtDoneFailed_Val_read/1 -> Subsystem/5(isAcsMdExtDoneFailed_Val_read)
  isAcsMdExtDoneOK_Val_read/1 -> Subsystem/6(isAcsMdExtDoneOK_Val_read)
  isINTMDoneFailed_Val_read/1 -> Subsystem/7(isINTMDoneFailed_Val_read)
  isINTMDoneOK_Val_read/1 -> Subsystem/8(isINTMDoneOK_Val_read)
  isINTMRDoneFailed_Val_read/1 -> Subsystem/9(isINTMRDoneFailed_Val_read)
  isINTMRDoneOK_Val_read/1 -> Subsystem/10(isINTMRDoneOK_Val_read)
  isLfFamlyDoneFailed_Val_read/1 -> Subsystem/11(isLfFamlyDoneFailed_Val_read)
  isLfFamlyDoneOK_Val_read/1 -> Subsystem/12(isLfFamlyDoneOK_Val_read)
  isLfLugDoneFailed_Val_read/1 -> Subsystem/13(isLfLugDoneFailed_Val_read)
  isLfLugDoneOK_Val_read/1 -> Subsystem/14(isLfLugDoneOK_Val_read)
  isLfLyDoneFailed_Val_read/1 -> Subsystem/15(isLfLyDoneFailed_Val_read)
  isLfLyDoneOK_Val_read/1 -> Subsystem/16(isLfLyDoneOK_Val_read)
  isLfRecoveryDoneFailed_Val_read/1 -> Subsystem/17(isLfRecoveryDoneFailed_Val_read)
  isLfRecoveryDoneOK_Val_read/1 -> Subsystem/18(isLfRecoveryDoneOK_Val_read)
  isLfVipDoneFailed_Val_read/1 -> Subsystem/19(isLfVipDoneFailed_Val_read)
  isLfVipDoneOK_Val_read/1 -> Subsystem/20(isLfVipDoneOK_Val_read)
  isLgrstCloseLDoneFailed_Val_read/1 -> Subsystem/21(isLgrstCloseLDoneFailed_Val_read)
  isLgrstCloseLDoneOK_Val_read/1 -> Subsystem/22(isLgrstCloseLDoneOK_Val_read)
  isLgrstCloseRDoneFailed_Val_read/1 -> Subsystem/23(isLgrstCloseRDoneFailed_Val_read)
  isLgrstCloseRDoneOK_Val_read/1 -> Subsystem/24(isLgrstCloseRDoneOK_Val_read)
  isLgrstOpenLDoneFailed_Val_read/1 -> Subsystem/25(isLgrstOpenLDoneFailed_Val_read)
  isLgrstOpenLDoneOK_Val_read/1 -> Subsystem/26(isLgrstOpenLDoneOK_Val_read)
  isLgrstOpenRDoneFailed_Val_read/1 -> Subsystem/27(isLgrstOpenRDoneFailed_Val_read)
  isLgrstOpenRDoneOK_Val_read/1 -> Subsystem/28(isLgrstOpenRDoneOK_Val_read)
  isRfFamlyDoneFailed_Val_read/1 -> Subsystem/29(isRfFamlyDoneFailed_Val_read)
  isRfFamlyDoneOK_Val_read/1 -> Subsystem/30(isRfFamlyDoneOK_Val_read)
  isRtLugDoneFailed_Val_read/1 -> Subsystem/31(isRtLugDoneFailed_Val_read)
  isRtLugDoneOK_Val_read/1 -> Subsystem/32(isRtLugDoneOK_Val_read)
  isRtLyDoneFailed_Val_read/1 -> Subsystem/33(isRtLyDoneFailed_Val_read)
  isRtLyDoneOK_Val_read/1 -> Subsystem/34(isRtLyDoneOK_Val_read)
  isRtRecoveryDoneFailed_Val_read/1 -> Subsystem/35(isRtRecoveryDoneFailed_Val_read)
  isRtRecoveryDoneOK_Val_read/1 -> Subsystem/36(isRtRecoveryDoneOK_Val_read)
  isRtVipDoneFailed_Val_read/1 -> Subsystem/37(isRtVipDoneFailed_Val_read)
  isRtVipDoneOK_Val_read/1 -> Subsystem/38(isRtVipDoneOK_Val_read)
  R3LMdSeatOccupied_Val_read/1 -> Subsystem/39(R3LMdSeatOccupied_Val_read)
  R3RMdSeatOccupied_Val_read/1 -> Subsystem/40(R3RMdSeatOccupied_Val_read)
  SoftIntAcsEnty_Val_read/1 -> Subsystem/41(SoftIntAcsEnty_Val_read)
  SoftIntAcsExt_Val_read/1 -> Subsystem/42(SoftIntAcsExt_Val_read)
  SoftIntAllLug_Val_read/1 -> Subsystem/43(SoftIntAllLug_Val_read)
  SoftIntAllVip_Val_read/1 -> Subsystem/44(SoftIntAllVip_Val_read)
  SoftIntIntimacyRt_Val_read/1 -> Subsystem/45(SoftIntIntimacyRt_Val_read)
  SoftIntINTM_Val_read/1 -> Subsystem/46(SoftIntINTM_Val_read)
  SoftIntLfFamly_Val_read/1 -> Subsystem/47(SoftIntLfFamly_Val_read)
  SoftIntLfLug_Val_read/1 -> Subsystem/48(SoftIntLfLug_Val_read)
  SoftIntLfLy_Val_read/1 -> Subsystem/49(SoftIntLfLy_Val_read)
  SoftIntLfRcvy_Val_read/1 -> Subsystem/50(SoftIntLfRcvy_Val_read)
  SoftIntLfVip_Val_read/1 -> Subsystem/51(SoftIntLfVip_Val_read)
  SoftIntLgrstCloseLt_Val_read/1 -> Subsystem/52(SoftIntLgrstCloseLt_Val_read)
  SoftIntLgrstCloseRt_Val_read/1 -> Subsystem/53(SoftIntLgrstCloseRt_Val_read)
  SoftIntLgrstOpenLt_Val_read/1 -> Subsystem/54(SoftIntLgrstOpenLt_Val_read)
  SoftIntLgrstOpenRt_Val_read/1 -> Subsystem/55(SoftIntLgrstOpenRt_Val_read)
  SoftIntRtFamly_Val_read/1 -> Subsystem/56(SoftIntRtFamly_Val_read)
  SoftIntRtLug_Val_read/1 -> Subsystem/57(SoftIntRtLug_Val_read)
  SoftIntRtLy_Val_read/1 -> Subsystem/58(SoftIntRtLy_Val_read)
  SoftIntRtRcvy_Val_read/1 -> Subsystem/59(SoftIntRtRcvy_Val_read)
  SoftIntRtVip_Val_read/1 -> Subsystem/60(SoftIntRtVip_Val_read)
  StNumFlg_Is4s_read/1 -> Subsystem/81(StNumFlg_Is4s_read)
  StNumFlg_Is6s_read/1 -> Subsystem/82(StNumFlg_Is6s_read)
  StNumFlg_Is6s7s_read/1 -> Subsystem/83(StNumFlg_Is6s7s_read)
  StNumFlg_Is7s_read/1 -> Subsystem/84(StNumFlg_Is7s_read)
  SwIntAcsEnty_Val_read/1 -> Subsystem/61(SwIntAcsEnty_Val_read)
  SwIntAcsExt_Val_read/1 -> Subsystem/62(SwIntAcsExt_Val_read)
  SwIntAllLug_Val_read/1 -> Subsystem/63(SwIntAllLug_Val_read)
  SwIntAllVip_Val_read/1 -> Subsystem/64(SwIntAllVip_Val_read)
  SwIntIntimacyRt_Val_read/1 -> Subsystem/65(SwIntIntimacyRt_Val_read)
  SwIntINTM_Val_read/1 -> Subsystem/66(SwIntINTM_Val_read)
  SwIntLfFamly_Val_read/1 -> Subsystem/67(SwIntLfFamly_Val_read)
  SwIntLfLug_Val_read/1 -> Subsystem/68(SwIntLfLug_Val_read)
  SwIntLfLy_Val_read/1 -> Subsystem/69(SwIntLfLy_Val_read)
  SwIntLfRcvy_Val_read/1 -> Subsystem/70(SwIntLfRcvy_Val_read)
  SwIntLfVip_Val_read/1 -> Subsystem/71(SwIntLfVip_Val_read)
  SwIntLgrstCloseLt_Val_read/1 -> Subsystem/72(SwIntLgrstCloseLt_Val_read)
  SwIntLgrstCloseRt_Val_read/1 -> Subsystem/73(SwIntLgrstCloseRt_Val_read)
  SwIntLgrstOpenLt_Val_read/1 -> Subsystem/74(SwIntLgrstOpenLt_Val_read)
  SwIntLgrstOpenRt_Val_read/1 -> Subsystem/75(SwIntLgrstOpenRt_Val_read)
  SwIntRtFamly_Val_read/1 -> Subsystem/76(SwIntRtFamly_Val_read)
  SwIntRtLug_Val_read/1 -> Subsystem/77(SwIntRtLug_Val_read)
  SwIntRtLy_Val_read/1 -> Subsystem/78(SwIntRtLy_Val_read)
  SwIntRtRcvy_Val_read/1 -> Subsystem/79(SwIntRtRcvy_Val_read)
  SwIntRtVip_Val_read/1 -> Subsystem/80(SwIntRtVip_Val_read)
  Subsystem/1(MdXX_Rsp_Md1_Rsp_write) -> MdXX_Rsp_Md1_Rsp_write/1
  Subsystem/2(MdXX_Rsp_Md10_Rsp_write) -> MdXX_Rsp_Md10_Rsp_write/1
  Subsystem/3(MdXX_Rsp_Md11_Rsp_write) -> MdXX_Rsp_Md11_Rsp_write/1
  Subsystem/4(MdXX_Rsp_Md12_Rsp_write) -> MdXX_Rsp_Md12_Rsp_write/1
  Subsystem/5(MdXX_Rsp_Md13_Rsp_write) -> MdXX_Rsp_Md13_Rsp_write/1
  Subsystem/6(MdXX_Rsp_Md14_Rsp_write) -> MdXX_Rsp_Md14_Rsp_write/1
  Subsystem/7(MdXX_Rsp_Md15_Rsp_write) -> MdXX_Rsp_Md15_Rsp_write/1
  Subsystem/8(MdXX_Rsp_Md16_Rsp_write) -> MdXX_Rsp_Md16_Rsp_write/1
  Subsystem/9(MdXX_Rsp_Md17_Rsp_write) -> MdXX_Rsp_Md17_Rsp_write/1
  Subsystem/10(MdXX_Rsp_Md18_Rsp_write) -> MdXX_Rsp_Md18_Rsp_write/1
  Subsystem/11(MdXX_Rsp_Md19_Rsp_write) -> MdXX_Rsp_Md19_Rsp_write/1
  Subsystem/12(MdXX_Rsp_Md2_Rsp_write) -> MdXX_Rsp_Md2_Rsp_write/1
  Subsystem/13(MdXX_Rsp_Md20_Rsp_write) -> MdXX_Rsp_Md20_Rsp_write/1
  Subsystem/14(MdXX_Rsp_Md21_Rsp_write) -> MdXX_Rsp_Md21_Rsp_write/1
  Subsystem/15(MdXX_Rsp_Md22_Rsp_write) -> MdXX_Rsp_Md22_Rsp_write/1
  Subsystem/16(MdXX_Rsp_Md23_Rsp_write) -> MdXX_Rsp_Md23_Rsp_write/1
  Subsystem/17(MdXX_Rsp_Md24_Rsp_write) -> MdXX_Rsp_Md24_Rsp_write/1
  Subsystem/18(MdXX_Rsp_Md25_Rsp_write) -> MdXX_Rsp_Md25_Rsp_write/1
  Subsystem/19(MdXX_Rsp_Md26_Rsp_write) -> MdXX_Rsp_Md26_Rsp_write/1
  Subsystem/20(MdXX_Rsp_Md27_Rsp_write) -> MdXX_Rsp_Md27_Rsp_write/1
  Subsystem/21(MdXX_Rsp_Md28_Rsp_write) -> MdXX_Rsp_Md28_Rsp_write/1
  Subsystem/22(MdXX_Rsp_Md29_Rsp_write) -> MdXX_Rsp_Md29_Rsp_write/1
  Subsystem/23(MdXX_Rsp_Md3_Rsp_write) -> MdXX_Rsp_Md3_Rsp_write/1
  Subsystem/24(MdXX_Rsp_Md30_Rsp_write) -> MdXX_Rsp_Md30_Rsp_write/1
  Subsystem/25(MdXX_Rsp_Md31_Rsp_write) -> MdXX_Rsp_Md31_Rsp_write/1
  Subsystem/26(MdXX_Rsp_Md32_Rsp_write) -> MdXX_Rsp_Md32_Rsp_write/1
  Subsystem/27(MdXX_Rsp_Md4_Rsp_write) -> MdXX_Rsp_Md4_Rsp_write/1
  Subsystem/28(MdXX_Rsp_Md5_Rsp_write) -> MdXX_Rsp_Md5_Rsp_write/1
  Subsystem/29(MdXX_Rsp_Md6_Rsp_write) -> MdXX_Rsp_Md6_Rsp_write/1
  Subsystem/30(MdXX_Rsp_Md7_Rsp_write) -> MdXX_Rsp_Md7_Rsp_write/1
  Subsystem/31(MdXX_Rsp_Md8_Rsp_write) -> MdXX_Rsp_Md8_Rsp_write/1
  Subsystem/32(MdXX_Rsp_Md9_Rsp_write) -> MdXX_Rsp_Md9_Rsp_write/1
  Subsystem/33(MdXX_Quit32bit_Val_write) -> MdXX_Quit32bit_Val_write/1

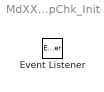
== system MdXX_RspChk/MdXX_RspChk_Init ==
  Event Listener : EventListener  EventName=reset
